simulink model "PID_Lab2"  (R2020a)
settings: Solver=VariableStepAuto  StartTime=0.0  StopTime=10  RelTol=1e-3
model workspace (MAT data in the model file):
  Ts = Simulink.Parameter
  Ts.Value = 0.005
  Ts.DataType = 'auto'
  Ts.Dimensions = [1 1]
undefined symbols (not defined in the file): DiscIntNeverNeededParam
libraries: simulink x2
settings Model: Creator=Lenovo  LastModifiedBy=Lenovo

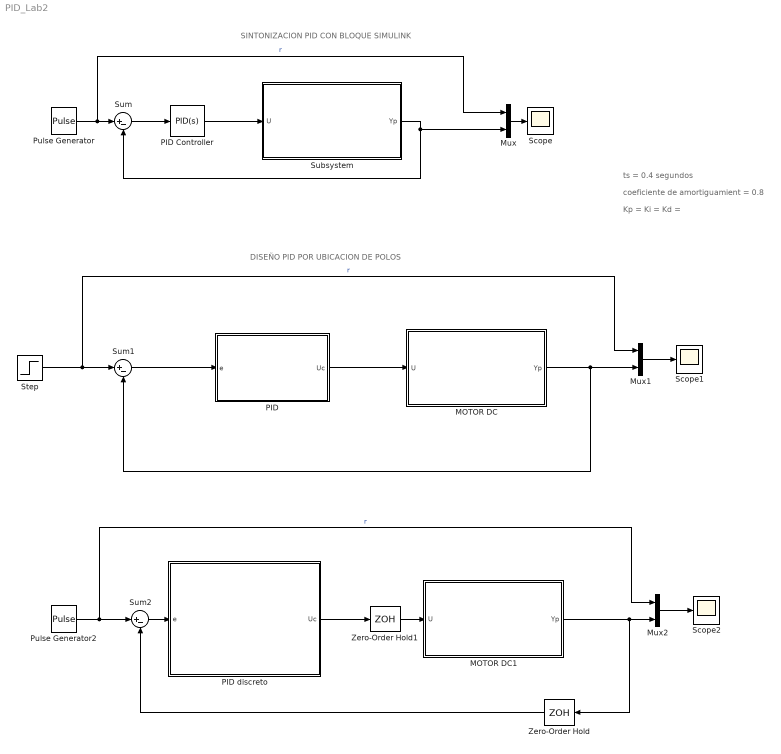
== system PID_Lab2 ==
  note: Kp =
      | Ki =
      | Kd =
  note: coeficiente de amortiguamient = 0.8
  note: ts = 0.4 segundos
  note: DISEÑO PID POR UBICACION DE POLOS
  note: SINTONIZACION PID CON BLOQUE SIMULINK
  MOTOR DC : Subsystem
  MOTOR DC1 : Subsystem
  Mux : Mux  Inputs=2
  Mux1 : Mux  Inputs=2
  Mux2 : Mux  Inputs=2
  PID : Subsystem
  PID Controller : simulink/Continuous/PID Controller  Controller=PID  Form=Parallel  TimeDomain=Continuous-time  UseExternalTs=off  SampleTime=-1  IntegratorMethod=Forward Euler  FilterMethod=Forward Euler  ControllerParametersSource=internal  P=0  I=0.295562586080053  D=0  UseFilter=on  N=100  TunerSelectOption=Transfer Function Based (PID Tuner App)  InitialConditionSource=internal  InitialConditionForIntegrator=0  InitialConditionForFilter=0  DifferentiatorICPrevScaledInput=0  ExternalReset=none  TrackingMode=off  Kt=1  LimitOutput=off  UpperSaturationLimit=inf  LowerSaturationLimit=-inf  LinearizeAsGain=on  AntiWindupMode=none  Kb=1  POutMin=[]  POutMax=[]  IOutMin=[]  IOutMax=[]  DOutMin=[]  DOutMax=[]  NOutMin=[]  NOutMax=[]  SumOutMin=[]  SumOutMax=[]  SaturationOutMin=[]  SaturationOutMax=[]  PParamMin=[]  PParamMax=[]  IParamMin=[]  IParamMax=[]  DParamMin=[]  DParamMax=[]  NParamMin=[]  NParamMax=[]  KbParamMin=[]  KbParamMax=[]  KtParamMin=[]  KtParamMax=[]  KbOutMin=[]  KbOutMax=[]  KtOutMin=[]  KtOutMax=[]  IntegratorOutMin=[]  IntegratorOutMax=[]  FilterOutMin=[]  FilterOutMax=[]  SumI1OutMin=[]  SumI1OutMax=[]  SumI2OutMin=[]  SumI2OutMax=[]  SumI3OutMin=[]  SumI3OutMax=[]  SumI4OutMin=[]  SumI4OutMax=[]  SumDOutMin=[]  SumDOutMax=[]  DifferentiatorOutMin=[]  DifferentiatorOutMax=[]  FilterDiffOutCoefMin=[]  FilterDiffOutCoefMax=[]  ReciprocalOutMin=[]  ReciprocalOutMax=[]  SumDenOutMin=[]  SumDenOutMax=[]  SumNumOutMin=[]  SumNumOutMax=[]  DivideOutMin=[]  DivideOutMax=[]  UdiffTsProdOutMin=[]  UdiffTsProdOutMax=[]  NTsProdOutMin=[]  NTsProdOutMax=[]  UintegralTsProdOutMin=[]  UintegralTsProdOutMax=[]  UngainTsProdOutMin=[]  UngainTsProdOutMax=[]  IntegratorContinuousStateAttributes=''  IntegratorStateMustResolveToSignalObject=off  IntegratorRTWStateStorageClass=Auto  FilterContinuousStateAttributes=''  FilterStateMustResolveToSignalObject=off  FilterRTWStateStorageClass=Auto  ParallelPVariant=InternalParameters  IdealPVariant=Disabled  IVariant=InternalParameters  DVariant=InternalParameters  IntegratorVariant=Continuous  SatVariant=Disabled  AWVariant=Passthrough  PCopyVariant=Disabled  TRVariant=Disabled  FdbkBlocksVariant=Forward  IdealPFdbkVariant=Disabled  SatFdbkVariant=Disabled  DerivativeFilterVariant=ContFilter  NVariant=InternalParameters  NCopyVariant=Disabled  FilterICVariant=InternalICsFilter  IntegratorICVariant=InternalICs  ExternalResetVariant=Disabled  TRSumVariant=Passthrough  SumFdbkVariant=Disabled  SumVariant=Sum_PID  TsampFilterVariant=InternalTs  TsampNgainVariant=Passthrough  TsampIntegralVariant=Passthrough
  PID discreto : Subsystem
  Pulse Generator : DiscretePulseGenerator  PulseType=Time based  Amplitude=3.14  Period=10  PulseWidth=50
  Pulse Generator2 : DiscretePulseGenerator  PulseType=Time based  Amplitude=3.14  Period=5  PulseWidth=50
  Scope : Scope
  Scope1 : Scope
  Scope2 : Scope
  Step : Step  SampleTime=0
  Subsystem : Subsystem
  Sum : Sum  Inputs=|+-
  Sum1 : Sum  Inputs=|+-
  Sum2 : Sum  Inputs=|+-
  Zero-Order Hold : ZeroOrderHold  SampleTime=Ts
  Zero-Order Hold1 : ZeroOrderHold  SampleTime=Ts
  wires:
  PID Controller/1 -> Subsystem/1(U)
  Sum/1 -> PID Controller/1
  Subsystem/1(Yp) -> Mux/2, Sum/2
  Mux/1 -> Scope/1
  Pulse Generator/1 -> Mux/1, Sum/1  "r"
  PID/1(Uc) -> MOTOR DC/1(U)
  Sum1/1 -> PID/1(e)
  Step/1 -> Mux1/1, Sum1/1  "r"
  MOTOR DC/1(Yp) -> Mux1/2, Sum1/2
  Mux1/1 -> Scope1/1
  Sum2/1 -> PID discreto/1(e)
  Pulse Generator2/1 -> Mux2/1, Sum2/1  "r"
  Mux2/1 -> Scope2/1
  MOTOR DC1/1(Yp) -> Zero-Order Hold/1, Mux2/2
  Zero-Order Hold1/1 -> MOTOR DC1/1(U)
  PID discreto/1(Uc) -> Zero-Order Hold1/1
  Zero-Order Hold/1 -> Sum2/2

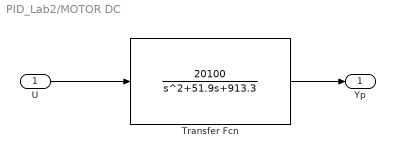
== system PID_Lab2/MOTOR DC ==
  U : Inport
  Transfer Fcn : TransferFcn  Numerator=[20100]  Denominator="[1   51.9  913.3]"
  Yp : Outport
  wires:
  Transfer Fcn/1 -> Yp/1
  U/1 -> Transfer Fcn/1

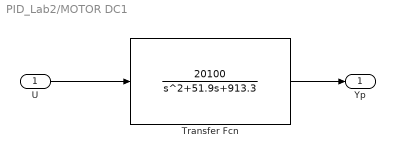
== system PID_Lab2/MOTOR DC1 ==
  U : Inport
  Transfer Fcn : TransferFcn  Numerator=[20100]  Denominator="[1   51.9  913.3]"
  Yp : Outport
  wires:
  Transfer Fcn/1 -> Yp/1
  U/1 -> Transfer Fcn/1

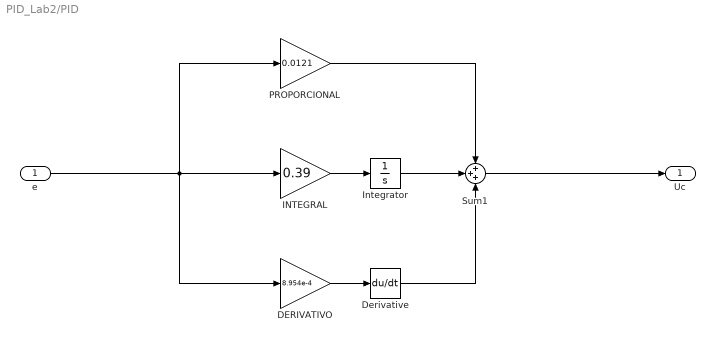
== system PID_Lab2/PID ==
  e : Inport
  DERIVATIVO : Gain  Gain=8.954e-4
  Derivative : Derivative
  INTEGRAL : Gain  Gain=0.39
  Integrator : Integrator
  PROPORCIONAL : Gain  Gain=0.0121
  Sum1 : Sum  Inputs=+++
  Uc : Outport
  wires:
  Sum1/1 -> Uc/1
  INTEGRAL/1 -> Integrator/1
  Integrator/1 -> Sum1/2
  e/1 -> DERIVATIVO/1, INTEGRAL/1, PROPORCIONAL/1
  DERIVATIVO/1 -> Derivative/1
  PROPORCIONAL/1 -> Sum1/1
  Derivative/1 -> Sum1/3

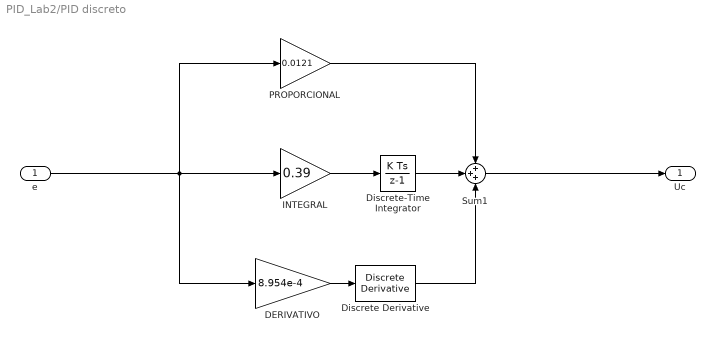
== system PID_Lab2/PID discreto ==
  e : Inport
  DERIVATIVO : Gain  Gain=8.954e-4
  Discrete Derivative : simulink/Discrete/Discrete Derivative  gainval=1.0  ICPrevScaledInput=0.0  OutMin=[]  OutMax=[]  OutDataType=fixdt(1, 16)  OutScaling=2^-10  DoSatur=off
  Discrete-Time Integrator : DiscreteIntegrator  SampleTime=Ts  ICPrevOutput=DiscIntNeverNeededParam  ICPrevScaledInput=DiscIntNeverNeededParam
  INTEGRAL : Gain  Gain=0.39
  PROPORCIONAL : Gain  Gain=0.0121
  Sum1 : Sum  Inputs=+++
  Uc : Outport
  wires:
  Sum1/1 -> Uc/1
  INTEGRAL/1 -> Discrete-Time Integrator/1
  Discrete-Time Integrator/1 -> Sum1/2
  e/1 -> DERIVATIVO/1, INTEGRAL/1, PROPORCIONAL/1
  DERIVATIVO/1 -> Discrete Derivative/1
  PROPORCIONAL/1 -> Sum1/1
  Discrete Derivative/1 -> Sum1/3

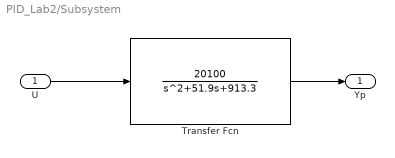
== system PID_Lab2/Subsystem ==
  U : Inport
  Transfer Fcn : TransferFcn  Numerator=[20100]  Denominator="[1   51.9  913.3]"
  Yp : Outport
  wires:
  Transfer Fcn/1 -> Yp/1
  U/1 -> Transfer Fcn/1
